simulink model "sim_att_dist_obs_tcyb"  (R2020a)
settings: Solver=ode4  StartTime=0.0  StopTime=30.0  FixedStep=0.01  RelTol=1e-3
values from neighbouring files (symbols this model uses):
  beta_Phi_1 = pp0 * cal_frac_squ( 3, p_p0_plus_1, q_p0_plus_1 )                          * cal_frac_squ( eps_s_bar / pi, p_p0_min_2, q_p0_min_2 )                          / ( 2 * ( 2 * pp0 - 1 ) * tanh( gamma0 * ( eps_s_bar / pi ) / 2 ) )                          - ( cal_frac_squ( 3, p_p0_plus_1, q_p0_plus_1 ) * gamma0 / ( 4 * ( 2 * pp0 -1 ) ) )                          * cal_frac_squ( eps_s_bar / pi, p_p0_min_ ...(+136 chars)    [init_att_dist_obs_tcyb.m]
  beta_Phi_2 = ( 1 - pp0 ) * cal_frac_squ( 3, p_p0_plus_1, q_p0_plus_1 )                          / ( 2 * ( 1 - 2 * pp0 ) * cal_frac_squ( eps_s_bar / pi, p_p0_0, q_p0_0 ) * tanh( gamma0 * ( eps_s_bar / pi ) / 2 ) )                          - ( cal_frac_squ( 3, p_p0_plus_1, q_p0_plus_1 ) * gamma0 / ( 4 * ( 1 - 2 * pp0 ) ) )                          * cal_frac_squ( eps_s_bar / pi, p_1_min_p0, q_1_min_p0 )          ...(+112 chars)    [init_att_dist_obs_tcyb.m]
  c1_diff_ui = diag([25; 30; 20])    [init_att_dist_obs_tcyb.m]
  c2_diff_ui = diag([50; 50; 10])    [init_att_dist_obs_tcyb.m]
  c3_diff_ui = diag([15; 15; 10])    [init_att_dist_obs_tcyb.m]
  c_w_1 = diag( [20; 15; 15] )    [init_att_dist_obs_tcyb.m]
  c_w_2 = diag( [20; 15; 15] )    [init_att_dist_obs_tcyb.m]
  c_w_3 = diag( [2; 2; 2] )    [init_att_dist_obs_tcyb.m]
  cS0 = diag( [4.5; 4.5; 4.5] )    [init_att_dist_obs_tcyb.m]
  dw_aa_t = 0.2 * ones(3, 5) + ( 1.0 - 0.2 ) * rand(3, 5)    [init_att_dist_obs_tcyb.m]
  dw_ff_t = [ 0.4 * ones(1, 5) + ( 1.0 - 0.4 ) * rand(1, 5);                      0.4 * ones(1, 5) + ( 1.0 - 0.4 ) * rand(1, 5);                      0.2 * ones(1, 5) + ( 0.6 - 0.2 ) * rand(1, 5) ]    [init_att_dist_obs_tcyb.m]
  dw_phi_t = ( - pi / 2 ) * ones(3, 5) + ( pi / 2 - ( - pi / 2 ) ) * rand(3, 5)    [init_att_dist_obs_tcyb.m]
  dwci_init = zeros(3,5)    [init_att_dist_obs_tcyb.m]
  eps_s_bar_div_pi = eps_s_bar / pi    (= 0.03)    [init_att_dist_obs_tcyb.m]
  gamma0 = 20    [init_att_dist_obs_tcyb.m]
  Ji = zeros(3,3,NF)    [init_att_dist_obs_tcyb.m]
  k_J_0 = diag( [1; 1; 1] )    [init_att_dist_obs_tcyb.m]
  Krw = diag([50; 50; 50])    [init_att_dist_obs_tcyb.m]
  Lamd_diff_ui = 0.8    [init_att_dist_obs_tcyb.m]
  mu_c_theta = 100    [init_att_dist_obs_tcyb.m]
  pos0 = zeros(3, 1)    [init_att_dist_obs_tcyb.m]
  pp0 = 8 / 11    (= 0.727272727273)    [init_att_dist_obs_tcyb.m]
  PZ0 = P0(3)    [init_att_dist_obs_tcyb.m]
  PZ1 = 10    [init_att_dist_obs_tcyb.m]
  Qci_init = repmat([1;0;0;0],1,NF)    [init_att_dist_obs_tcyb.m]
  R0 = 4    [init_att_dist_obs_tcyb.m]
  R1 = 8    [init_att_dist_obs_tcyb.m]
  Rci_init = zeros(3,3,NF)    [init_att_dist_obs_tcyb.m]
  Ri_init = zeros(3,3,NF)    [init_att_dist_obs_tcyb.m]
  Rx2 = 10    [init_att_dist_obs_tcyb.m]
  Ry2 = 6    [init_att_dist_obs_tcyb.m]
  Rz2 = 4    [init_att_dist_obs_tcyb.m]
  T0 = 0    [init_att_dist_obs_tcyb.m]
  T1 = tseq1    (= 10)    [init_att_dist_obs_tcyb.m]
  T2 = tseq1 + tseq12 + tseq2    (= 30)    [init_att_dist_obs_tcyb.m]
  thr_p_plus_1 = cal_frac_squ( 3, p_p0_plus_1, q_p0_plus_1 )    [init_att_dist_obs_tcyb.m]
  ui_init = zeros(3,NF)    [init_att_dist_obs_tcyb.m]
  vel0 = zeros(3, 1)    [init_att_dist_obs_tcyb.m]
  wci_init = zeros(3,5)    [init_att_dist_obs_tcyb.m]
  zeta_diff_ui = 0.05    [init_att_dist_obs_tcyb.m]
undefined symbols (not defined in the file or in its folder): cal_frac_squ, p_2_p0, p_beta_w_1, p_beta_w_2, p_p0_min_1, p_p0_plus_1, q_2_p0, q_beta_w_1, q_beta_w_2, q_p0_min_1, q_p0_plus_1, Qei_init, Qi_init, Rei_init, V_Phi_Rei_init, wei_init, wi_init
(part 2 of 4)

== matlab function sim_att_dist_obs_tcyb/Qei dynam agent 1 ==
  data: Qei_vec input; dQei_1 output; wei_vec input
function dQei_1 = fcn(Qei_vec, wei_vec)
%%%% 更新四元数误差微分方程
iiuav = 1;

wei = wei_vec(:,iiuav);
thetaei = Qei_vec(1,iiuav);
qei = Qei_vec(2:4,iiuav);

GammaQei = zeros(4,3);
GammaQei(1,:) = -(qei');
GammaQei(2:4,:) = thetaei*eye(3,3) + cal_askew_mat(qei);
dQei_1 = (1/2)*GammaQei*wei;

end

== matlab function sim_att_dist_obs_tcyb/cal d_theta_hat1 ==
  data: c1 input; d_ui_hat output; d_dui_hat output; d_d2ui_hat output; c2 input; c3 input; chi_t input; ui_sig_1 input; ui_sig_2 input; ui_sig_3 input; ui_sig_4 input; ui_sig_5 input; ui_sig_6 input; dui_hat input; d2ui_hat input
function [d_ui_hat, d_dui_hat, d_d2ui_hat] = fcn(c1, c2, c3, chi_t, ui_sig_1, ui_sig_2, ui_sig_3, ...
                                                                                        ui_sig_4, ui_sig_5, ui_sig_6, dui_hat, d2ui_hat)
d_d2ui_hat = -chi_t .* c1 * ui_sig_1(:) - (1 - chi_t) .* c1 * ui_sig_2(:);
d_dui_hat = -chi_t .* c2 * ui_sig_3(:) - (1 - chi_t) .* c2 * ui_sig_4(:) + d2ui_hat(:);
d_ui_hat = -chi_t .* c3 * ui_sig_5(:) - (1 - chi_t) .* c3 * ui_sig_6(:) + dui_hat(:);

== matlab function sim_att_dist_obs_tcyb/cal d_theta_hat2 ==
  data: c1 input; d_ui_hat output; d_dui_hat output; d_d2ui_hat output; c2 input; c3 input; chi_t input; ui_sig_1 input; ui_sig_2 input; ui_sig_3 input; ui_sig_4 input; ui_sig_5 input; ui_sig_6 input; dui_hat input; d2ui_hat input
function [d_ui_hat, d_dui_hat, d_d2ui_hat] = fcn(c1, c2, c3, chi_t, ui_sig_1, ui_sig_2, ui_sig_3, ...
                                                                                        ui_sig_4, ui_sig_5, ui_sig_6, dui_hat, d2ui_hat)
d_d2ui_hat = -chi_t .* c1 * ui_sig_1(:) - (1 - chi_t) .* c1 * ui_sig_2(:);
d_dui_hat = -chi_t .* c2 * ui_sig_3(:) - (1 - chi_t) .* c2 * ui_sig_4(:) + d2ui_hat(:);
d_ui_hat = -chi_t .* c3 * ui_sig_5(:) - (1 - chi_t) .* c3 * ui_sig_6(:) + dui_hat(:);

== matlab function sim_att_dist_obs_tcyb/cal d_theta_hat3 ==
  data: c1 input; d_ui_hat output; d_dui_hat output; d_d2ui_hat output; c2 input; c3 input; chi_t input; ui_sig_1 input; ui_sig_2 input; ui_sig_3 input; ui_sig_4 input; ui_sig_5 input; ui_sig_6 input; dui_hat input; d2ui_hat input
function [d_ui_hat, d_dui_hat, d_d2ui_hat] = fcn(c1, c2, c3, chi_t, ui_sig_1, ui_sig_2, ui_sig_3, ...
                                                                                        ui_sig_4, ui_sig_5, ui_sig_6, dui_hat, d2ui_hat)
d_d2ui_hat = -chi_t .* c1 * ui_sig_1(:) - (1 - chi_t) .* c1 * ui_sig_2(:);
d_dui_hat = -chi_t .* c2 * ui_sig_3(:) - (1 - chi_t) .* c2 * ui_sig_4(:) + d2ui_hat(:);
d_ui_hat = -chi_t .* c3 * ui_sig_5(:) - (1 - chi_t) .* c3 * ui_sig_6(:) + dui_hat(:);

== matlab function sim_att_dist_obs_tcyb/cal d_theta_hat4 ==
  data: c1 input; d_ui_hat output; d_dui_hat output; d_d2ui_hat output; c2 input; c3 input; chi_t input; ui_sig_1 input; ui_sig_2 input; ui_sig_3 input; ui_sig_4 input; ui_sig_5 input; ui_sig_6 input; dui_hat input; d2ui_hat input
function [d_ui_hat, d_dui_hat, d_d2ui_hat] = fcn(c1, c2, c3, chi_t, ui_sig_1, ui_sig_2, ui_sig_3, ...
                                                                                        ui_sig_4, ui_sig_5, ui_sig_6, dui_hat, d2ui_hat)
d_d2ui_hat = -chi_t .* c1 * ui_sig_1(:) - (1 - chi_t) .* c1 * ui_sig_2(:);
d_dui_hat = -chi_t .* c2 * ui_sig_3(:) - (1 - chi_t) .* c2 * ui_sig_4(:) + d2ui_hat(:);
d_ui_hat = -chi_t .* c3 * ui_sig_5(:) - (1 - chi_t) .* c3 * ui_sig_6(:) + dui_hat(:);

== matlab function sim_att_dist_obs_tcyb/process velocity ==
  data: T0 input; T1 input; T2 input; PZ0 input; PZ1 input; R0 input; R1 input; Rx2 input; Ry2 input; Rz2 input; t input; V_init_out output
function V_init_out = fcn(T0, T1, T2, PZ0, PZ1, R0, R1, Rx2, Ry2, Rz2, t)
V_init_out = zeros(3, 1);
if t < T1 + 1e-05
    V_init_out(1, 1) = ( cos( ( 2 * pi * ( t - T0 ) ) / ( T0 - T1 ) ) * ( R0 - R1 ) ) / ( T0 - T1 ) ...
                                    - ( 2 * pi * sin( ( 2 * pi * ( t - T0 ) ) / ( T0 - T1 ) ) * ( R0 + ( ( R0 - R1 ) * ( t - T0 ) ) / ( T0 - T1 ) ) ) / ( T0 - T1 );
    V_init_out(2, 1) = ( sin( ( 2 * pi * ( t - T0 ) ) / ( T0 - T1 ) ) * ( R0 - R1 ) ) / ( T0 - T1 ) ...
                                    + ( 2 * pi * cos( ( 2 * pi * ( t - T0 ) ) / ( T0 - T1 ) ) * ( R0 + ( ( R0 - R1 ) * ( t - T0 ) ) / ( T0 - T1 ) ) ) / ( T0 - T1 );
    V_init_out(3, 1) = ( PZ0 - PZ1 ) / ( T0 - T1 );
else
    V_init_out(1, 1) = ( 2 * Rx2 * pi * sin( ( 2 * pi * ( t - T1 ) ) / ( T1 - T2 ) ) ) / ( T1 - T2 );
    V_init_out(2, 1) = ( 4 * Ry2 * pi * cos( ( 4 * pi * ( t - T1 ) ) / ( T1 - T2 ) ) ) / ( T1 - T2 );
    V_init_out(3, 1) = - ( 4 * Rz2 * pi * cos( ( 4 * pi * ( t - T1 ) ) / ( T1 - T2 ) ) ) / ( T1 - T2 );
end

== matlab function sim_att_dist_obs_tcyb/cal divide pi ==
  data: x input; y output
function y = fcn(x)
y = x ./ pi;

== matlab function sim_att_dist_obs_tcyb/cal sig ==
  data: x input; z output; y input
function z = fcn(x, y)
z = x(:) .* sign(y(:));

== matlab function sim_att_dist_obs_tcyb/cal sig1 ==
  data: x input; z output; y input
function z = fcn(x, y)
z = x(:) .* sign(y(:));

== matlab function sim_att_dist_obs_tcyb/cal sig10 ==
  data: x input; z output; y input
function z = fcn(x, y)
z = x(:) .* sign(y(:));

== matlab function sim_att_dist_obs_tcyb/cal sig11 ==
  data: x input; z output; y input
function z = fcn(x, y)
z = x(:) .* sign(y(:));

== matlab function sim_att_dist_obs_tcyb/cal sig12 ==
  data: x input; z output; y input
function z = fcn(x, y)
z = x(:) .* sign(y(:));

== matlab function sim_att_dist_obs_tcyb/cal sig13 ==
  data: x input; z output; y input
function z = fcn(x, y)
z = x(:) .* sign(y(:));

== matlab function sim_att_dist_obs_tcyb/cal sig14 ==
  data: x input; z output; y input
function z = fcn(x, y)
z = x(:) .* sign(y(:));

== matlab function sim_att_dist_obs_tcyb/cal sig15 ==
  data: x input; z output; y input
function z = fcn(x, y)
z = x(:) .* sign(y(:));

== matlab function sim_att_dist_obs_tcyb/cal sig16 ==
  data: x input; z output; y input
function z = fcn(x, y)
z = x(:) .* sign(y(:));

== matlab function sim_att_dist_obs_tcyb/cal sig17 ==
  data: x input; z output; y input
function z = fcn(x, y)
z = x(:) .* sign(y(:));

== matlab function sim_att_dist_obs_tcyb/cal sig18 ==
  data: x input; z output; y input
function z = fcn(x, y)
z = x(:) .* sign(y(:));

== matlab function sim_att_dist_obs_tcyb/cal sig19 ==
  data: x input; z output; y input
function z = fcn(x, y)
z = x(:) .* sign(y(:));

== matlab function sim_att_dist_obs_tcyb/cal sig2 ==
  data: x input; z output; y input
function z = fcn(x, y)
z = x(:) .* sign(y(:));

== matlab function sim_att_dist_obs_tcyb/cal sig20 ==
  data: x input; z output; y input
function z = fcn(x, y)
z = x(:) .* sign(y(:));

== matlab function sim_att_dist_obs_tcyb/cal sig21 ==
  data: x input; z output; y input
function z = fcn(x, y)
z = x(:) .* sign(y(:));

== matlab function sim_att_dist_obs_tcyb/cal sig22 ==
  data: x input; z output; y input
function z = fcn(x, y)
z = x(:) .* sign(y(:));

== matlab function sim_att_dist_obs_tcyb/cal sig23 ==
  data: x input; z output; y input
function z = fcn(x, y)
z = x(:) .* sign(y(:));

== matlab function sim_att_dist_obs_tcyb/cal sig24 ==
  data: x input; z output; y input
function z = fcn(x, y)
z = x(:) .* sign(y(:));

== matlab function sim_att_dist_obs_tcyb/cal sig25 ==
  data: x input; z output; y input
function z = fcn(x, y)
z = x(:) .* sign(y(:));

== matlab function sim_att_dist_obs_tcyb/cal sig26 ==
  data: x input; z output; y input
function z = fcn(x, y)
z = x(:) .* sign(y(:));

== matlab function sim_att_dist_obs_tcyb/Qei dynam agent 2 ==
  data: Qei_vec input; dQei_2 output; wei_vec input
function dQei_2 = fcn(Qei_vec, wei_vec)
%%%% 更新四元数误差微分方程
iiuav = 2;

wei = wei_vec(:,iiuav);
thetaei = Qei_vec(1,iiuav);
qei = Qei_vec(2:4,iiuav);

GammaQei = zeros(4,3);
GammaQei(1,:) = -(qei');
GammaQei(2:4,:) = thetaei*eye(3,3) + cal_askew_mat(qei);
dQei_2 = (1/2)*GammaQei*wei;

end

== matlab function sim_att_dist_obs_tcyb/cal sig27 ==
  data: x input; z output; y input
function z = fcn(x, y)
z = x(:) .* sign(y(:));

== matlab function sim_att_dist_obs_tcyb/cal sig28 ==
  data: x input; z output; y input
function z = fcn(x, y)
z = x(:) .* sign(y(:));

== matlab function sim_att_dist_obs_tcyb/cal sig29 ==
  data: x input; z output; y input
function z = fcn(x, y)
z = x(:) .* sign(y(:));

== matlab function sim_att_dist_obs_tcyb/cal sig3 ==
  data: x input; z output; y input
function z = fcn(x, y)
z = x(:) .* sign(y(:));

== matlab function sim_att_dist_obs_tcyb/cal sig4 ==
  data: x input; z output; y input
function z = fcn(x, y)
z = x(:) .* sign(y(:));

== matlab function sim_att_dist_obs_tcyb/cal sig5 ==
  data: x input; z output; y input
function z = fcn(x, y)
z = x(:) .* sign(y(:));

== matlab function sim_att_dist_obs_tcyb/cal sig6 ==
  data: x input; z output; y input
function z = fcn(x, y)
z = x(:) .* sign(y(:));

== matlab function sim_att_dist_obs_tcyb/cal sig7 ==
  data: x input; z output; y input
function z = fcn(x, y)
z = x(:) .* sign(y(:));

== matlab function sim_att_dist_obs_tcyb/cal sig8 ==
  data: x input; z output; y input
function z = fcn(x, y)
z = x(:) .* sign(y(:));

== matlab function sim_att_dist_obs_tcyb/cal sig9 ==
  data: x input; z output; y input
function z = fcn(x, y)
z = x(:) .* sign(y(:));

== matlab function sim_att_dist_obs_tcyb/combine dw_hat1 ==
  data: eps_w_hat_1 input; eps_w_hat_2 input; eps_w_hat_3 input; eps_w_hat_4 input; eps_w_hat_5 input; eps_w_hat_vec output
function eps_w_hat_vec  = fcn(eps_w_hat_1, eps_w_hat_2, eps_w_hat_3, eps_w_hat_4, eps_w_hat_5)
%%%% 合并扰动观测值dw_hat
eps_w_hat_vec = [eps_w_hat_1(:), eps_w_hat_2(:), eps_w_hat_3(:), eps_w_hat_4(:), eps_w_hat_5(:)];

== matlab function sim_att_dist_obs_tcyb/cal taui agent 1 ==
  data: c_w_1 input; c_w_2 input; c_w_3 input; k_J_0 input; tau_1 output; Ji input; Si_vec input; dw_hat_vec input; Fi_S_vec input; theta_Si_beta_w_1_vec input; theta_Si_beta_w_2_vec input
function tau_1 = fcn(c_w_1, c_w_2, c_w_3, k_J_0, Ji, Si_vec, dw_hat_vec, ...
                                        Fi_S_vec, theta_Si_beta_w_1_vec, theta_Si_beta_w_2_vec)
%%%% 计算用于姿态控制的驱动力矩控制输入
iiuav = 1;
tau_1 = -c_w_1 * theta_Si_beta_w_1_vec(:,iiuav) - c_w_2 * theta_Si_beta_w_2_vec(:,iiuav) - c_w_3 * Si_vec(:,iiuav) ...
                - dw_hat_vec(:,iiuav) - k_J_0 * inv( Ji(:,:,iiuav) ) * Fi_S_vec(:,iiuav);
end

== matlab function sim_att_dist_obs_tcyb/cal taui agent 2 ==
  data: c_w_1 input; c_w_2 input; c_w_3 input; k_J_0 input; tau_2 output; Ji input; Si_vec input; dw_hat_vec input; Fi_S_vec input; theta_Si_beta_w_1_vec input; theta_Si_beta_w_2_vec input
function tau_2 = fcn(c_w_1, c_w_2, c_w_3, k_J_0, Ji, Si_vec, dw_hat_vec, ...
                                        Fi_S_vec, theta_Si_beta_w_1_vec, theta_Si_beta_w_2_vec)
%%%% 计算用于姿态控制的驱动力矩控制输入
iiuav = 2;
tau_2 = -c_w_1 * theta_Si_beta_w_1_vec(:,iiuav) - c_w_2 * theta_Si_beta_w_2_vec(:,iiuav) - c_w_3 * Si_vec(:,iiuav) ...
                - dw_hat_vec(:,iiuav) - k_J_0 * inv( Ji(:,:,iiuav) ) * Fi_S_vec(:,iiuav);
end

== matlab function sim_att_dist_obs_tcyb/cal taui agent 3 ==
  data: c_w_1 input; c_w_2 input; c_w_3 input; k_J_0 input; tau_3 output; Ji input; Si_vec input; dw_hat_vec input; Fi_S_vec input; theta_Si_beta_w_1_vec input; theta_Si_beta_w_2_vec input
function tau_3 = fcn(c_w_1, c_w_2, c_w_3, k_J_0, Ji, Si_vec, dw_hat_vec, ...
                                        Fi_S_vec, theta_Si_beta_w_1_vec, theta_Si_beta_w_2_vec)
%%%% 计算用于姿态控制的驱动力矩控制输入
iiuav = 3;
tau_3 = -c_w_1 * theta_Si_beta_w_1_vec(:,iiuav) - c_w_2 * theta_Si_beta_w_2_vec(:,iiuav) - c_w_3 * Si_vec(:,iiuav) ...
                - dw_hat_vec(:,iiuav) - k_J_0 * inv( Ji(:,:,iiuav) ) * Fi_S_vec(:,iiuav);
end

== matlab function sim_att_dist_obs_tcyb/cal taui agent 4 ==
  data: c_w_1 input; c_w_2 input; c_w_3 input; k_J_0 input; tau_4 output; Ji input; Si_vec input; dw_hat_vec input; Fi_S_vec input; theta_Si_beta_w_1_vec input; theta_Si_beta_w_2_vec input
function tau_4 = fcn(c_w_1, c_w_2, c_w_3, k_J_0, Ji, Si_vec, dw_hat_vec, ...
                                        Fi_S_vec, theta_Si_beta_w_1_vec, theta_Si_beta_w_2_vec)
%%%% 计算用于姿态控制的驱动力矩控制输入
iiuav = 4;
tau_4 = -c_w_1 * theta_Si_beta_w_1_vec(:,iiuav) - c_w_2 * theta_Si_beta_w_2_vec(:,iiuav) - c_w_3 * Si_vec(:,iiuav) ...
                - dw_hat_vec(:,iiuav) - k_J_0 * inv( Ji(:,:,iiuav) ) * Fi_S_vec(:,iiuav);
end

== matlab function sim_att_dist_obs_tcyb/cal taui agent 5 ==
  data: c_w_1 input; c_w_2 input; c_w_3 input; k_J_0 input; tau_5 output; Ji input; Si_vec input; dw_hat_vec input; Fi_S_vec input; theta_Si_beta_w_1_vec input; theta_Si_beta_w_2_vec input
function tau_5 = fcn(c_w_1, c_w_2, c_w_3, k_J_0, Ji, Si_vec, dw_hat_vec, ...
                                        Fi_S_vec, theta_Si_beta_w_1_vec, theta_Si_beta_w_2_vec)
%%%% 计算用于姿态控制的驱动力矩控制输入
iiuav = 5;
tau_5 = -c_w_1 * theta_Si_beta_w_1_vec(:,iiuav) - c_w_2 * theta_Si_beta_w_2_vec(:,iiuav) - c_w_3 * Si_vec(:,iiuav) ...
                - dw_hat_vec(:,iiuav) - k_J_0 * inv( Ji(:,:,iiuav) ) * Fi_S_vec(:,iiuav);
end

== matlab function sim_att_dist_obs_tcyb/cal theta_Si_beta_w agent 1 ==
  data: mu_c_theta input; Si_squ_beta_w_1_vec input; theta_Si_beta_w_1_node_1 output; Si_squ_beta_w_2_vec input; Si_vec input; theta_Si_beta_w_2_node_1 output
function [theta_Si_beta_w_1_node_1, theta_Si_beta_w_2_node_1] = fcn(mu_c_theta, Si_squ_beta_w_1_vec, Si_squ_beta_w_2_vec, Si_vec)
%%%% 计算平滑递增函数
iiuav = 1;
theta_Si_beta_w_1_node_1 = Si_squ_beta_w_1_vec(:, iiuav) .* ( -1 + 2 ./ ( 1 + exp( -mu_c_theta .* Si_vec(:,iiuav) ) ) );
theta_Si_beta_w_2_node_1 = Si_squ_beta_w_2_vec(:, iiuav) .* ( -1 + 2 ./ ( 1 + exp( -mu_c_theta .* Si_vec(:,iiuav) ) ) );

== matlab function sim_att_dist_obs_tcyb/cal theta_Si_beta_w agent 2 ==
  data: mu_c_theta input; Si_squ_beta_w_1_vec input; theta_Si_beta_w_1_node_2 output; Si_squ_beta_w_2_vec input; Si_vec input; theta_Si_beta_w_2_node_2 output
function [theta_Si_beta_w_1_node_2, theta_Si_beta_w_2_node_2] = fcn(mu_c_theta, Si_squ_beta_w_1_vec, Si_squ_beta_w_2_vec, Si_vec)
%%%% 计算平滑递增函数
iiuav = 2;
theta_Si_beta_w_1_node_2 = Si_squ_beta_w_1_vec(:, iiuav) .* ( -1 + 2 ./ ( 1 + exp( -mu_c_theta .* Si_vec(:,iiuav) ) ) );
theta_Si_beta_w_2_node_2 = Si_squ_beta_w_2_vec(:, iiuav) .* ( -1 + 2 ./ ( 1 + exp( -mu_c_theta .* Si_vec(:,iiuav) ) ) );

== matlab function sim_att_dist_obs_tcyb/cal theta_Si_beta_w agent 3 ==
  data: mu_c_theta input; Si_squ_beta_w_1_vec input; theta_Si_beta_w_1_node_3 output; Si_squ_beta_w_2_vec input; Si_vec input; theta_Si_beta_w_2_node_3 output
function [theta_Si_beta_w_1_node_3, theta_Si_beta_w_2_node_3] = fcn(mu_c_theta, Si_squ_beta_w_1_vec, Si_squ_beta_w_2_vec, Si_vec)
%%%% 计算平滑递增函数
iiuav = 3;
theta_Si_beta_w_1_node_3 = Si_squ_beta_w_1_vec(:, iiuav) .* ( -1 + 2 ./ ( 1 + exp( -mu_c_theta .* Si_vec(:,iiuav) ) ) );
theta_Si_beta_w_2_node_3 = Si_squ_beta_w_2_vec(:, iiuav) .* ( -1 + 2 ./ ( 1 + exp( -mu_c_theta .* Si_vec(:,iiuav) ) ) );

== matlab function sim_att_dist_obs_tcyb/cal eps_w_hat agent 1 ==
  data: Ji input; Krw input; eps_w_hat_vec input; wi_vec input; d_eps_w_hat_1 output; taui_vec input
function d_eps_w_hat_1 = fcn(Ji, Krw, eps_w_hat_vec, wi_vec, taui_vec)
%%%% 计算扰动观测中间变量
iiuav = 1;
d_eps_w_hat_1 = -Krw * inv(Ji(:,:,iiuav)) * ( eps_w_hat_vec(:,iiuav) + taui_vec(:,iiuav) ...
                                                                        - cal_askew_mat(wi_vec(:,iiuav)) * Ji(:,:,iiuav) * wi_vec(:,iiuav) ) ...
                                                                        - Krw * Krw * inv(Ji(:,:,iiuav)) * wi_vec(:,iiuav);

== matlab function sim_att_dist_obs_tcyb/cal theta_Si_beta_w agent 4 ==
  data: mu_c_theta input; Si_squ_beta_w_1_vec input; theta_Si_beta_w_1_node_4 output; Si_squ_beta_w_2_vec input; Si_vec input; theta_Si_beta_w_2_node_4 output
function [theta_Si_beta_w_1_node_4, theta_Si_beta_w_2_node_4] = fcn(mu_c_theta, Si_squ_beta_w_1_vec, Si_squ_beta_w_2_vec, Si_vec)
%%%% 计算平滑递增函数
iiuav = 4;
theta_Si_beta_w_1_node_4 = Si_squ_beta_w_1_vec(:, iiuav) .* ( -1 + 2 ./ ( 1 + exp( -mu_c_theta .* Si_vec(:,iiuav) ) ) );
theta_Si_beta_w_2_node_4 = Si_squ_beta_w_2_vec(:, iiuav) .* ( -1 + 2 ./ ( 1 + exp( -mu_c_theta .* Si_vec(:,iiuav) ) ) );

== matlab function sim_att_dist_obs_tcyb/cal theta_Si_beta_w agent 5 ==
  data: mu_c_theta input; Si_squ_beta_w_1_vec input; theta_Si_beta_w_1_node_5 output; Si_squ_beta_w_2_vec input; Si_vec input; theta_Si_beta_w_2_node_5 output
function [theta_Si_beta_w_1_node_5, theta_Si_beta_w_2_node_5] = fcn(mu_c_theta, Si_squ_beta_w_1_vec, Si_squ_beta_w_2_vec, Si_vec)
%%%% 计算平滑递增函数
iiuav = 5;
theta_Si_beta_w_1_node_5 = Si_squ_beta_w_1_vec(:, iiuav) .* ( -1 + 2 ./ ( 1 + exp( -mu_c_theta .* Si_vec(:,iiuav) ) ) );
theta_Si_beta_w_2_node_5 = Si_squ_beta_w_2_vec(:, iiuav) .* ( -1 + 2 ./ ( 1 + exp( -mu_c_theta .* Si_vec(:,iiuav) ) ) );

== matlab function sim_att_dist_obs_tcyb/cal wci dwci agent 1 ==
  data: ui_vec input; wci output; duihat_vec input; d2uihat_vec input; Rci_mat input; dwci output
function [wci, dwci] = fcn(ui_vec, duihat_vec, d2uihat_vec, Rci_mat)
%%%% 计算姿态角速率指令及其导数

iiuav = 1;
ui = ui_vec(:,iiuav);
duihat = duihat_vec(:,iiuav);
d2uihat = d2uihat_vec(:,iiuav);
Rci = Rci_mat(:,:,iiuav);

ee1 = [1;0;0];
ee2 = [0;1;0];
ee3 = [0;0;1];
RciE3 = ui / norm(ui,2);
PiMat = eye(3,3) - ee3*(ee3');
dRciE3 = (1 / norm(ui,2))*Rci*PiMat*(Rci')*duihat;
Themat = [-RciE3(2)/(1+RciE3(3)),         -RciE3(1)/(1+RciE3(3)),       (RciE3(1)*RciE3(2))/((1+RciE3(3))^2); ...
                   2*RciE3(1)/(1+RciE3(3)),                0,                               1 - (RciE3(1)^2)/((1+RciE3(3))^2); ...
                               0                                       -1                                                        0                                   ];
wcxe3 = (1 / norm(ui,2))*PiMat*(Rci')*duihat;
wcxe2 = (1 / norm(ui,2))*(Rci')*Themat*Rci*PiMat*(Rci')*duihat;
wci = [-wcxe3(2); wcxe3(1); -wcxe2(1)];

TempMat1 = [0,                           -1/(1+RciE3(3)),                   (RciE3(2))/((1+RciE3(3))^2); ...
                       2/(1+RciE3(3)),                0,                               (-2*RciE3(1))/((1+RciE3(3))^2); ...
                       0,                                     0,                                                   0                             ];
TempMat2 = [-1/(1+RciE3(3)),              0,                               (RciE3(1))/((1+RciE3(3))^2); ...
                       0,                                     0,                                                   0                      ; ...
                       0,                                     0,                                                   0                             ];
TempMat3 = [(RciE3(2))/((1+RciE3(3))^2),                 (RciE3(1))/((1+RciE3(3))^2),       (-2*RciE3(1)*RciE3(2))/((1+RciE3(3))^3); ...
                       (-2*RciE3(1))/((1+RciE3(3))^2),                             0,                               (2*(RciE3(1)^2))/((1+RciE3(3))^3); ...
                        0,                                                                          0,                                                   0                             ];
dTheMat = TempMat1*dRciE3*(ee1') + TempMat2*dRciE3*(ee2') + TempMat3*dRciE3*(ee3');
wcix = cal_askew_mat(wci);
dRciT = -wcix*(Rci');
dwcxe3 = (1 / norm(ui,2))*PiMat*(dRciT*duihat+(Rci')*(d2uihat-(((ui')*duihat)/(norm(ui,2)^2))*duihat));
dwcxe2 = (1 / norm(ui,2))*((dRciT*Themat+(Rci')*dTheMat) ...
                *(Rci*PiMat*(Rci'))*duihat + (Rci')*Themat*(Rci*PiMat*(Rci'))*(d2uihat-(((ui')*duihat)/(norm(ui,2)^2))*duihat));
dwci = [-dwcxe3(2);  dwcxe3(1);  -dwcxe2(1)];

== matlab function sim_att_dist_obs_tcyb/cal wci dwci agent 2 ==
  data: ui_vec input; wci output; duihat_vec input; d2uihat_vec input; Rci_mat input; dwci output
function [wci, dwci] = fcn(ui_vec, duihat_vec, d2uihat_vec, Rci_mat)
%%%% 计算姿态角速率指令及其导数

iiuav = 2;
ui = ui_vec(:,iiuav);
duihat = duihat_vec(:,iiuav);
d2uihat = d2uihat_vec(:,iiuav);
Rci = Rci_mat(:,:,iiuav);

ee1 = [1;0;0];
ee2 = [0;1;0];
ee3 = [0;0;1];
RciE3 = ui / norm(ui,2);
PiMat = eye(3,3) - ee3*(ee3');
dRciE3 = (1 / norm(ui,2))*Rci*PiMat*(Rci')*duihat;
Themat = [-RciE3(2)/(1+RciE3(3)),         -RciE3(1)/(1+RciE3(3)),       (RciE3(1)*RciE3(2))/((1+RciE3(3))^2); ...
                   2*RciE3(1)/(1+RciE3(3)),                0,                               1 - (RciE3(1)^2)/((1+RciE3(3))^2); ...
                               0                                       -1                                                        0                                   ];
wcxe3 = (1 / norm(ui,2))*PiMat*(Rci')*duihat;
wcxe2 = (1 / norm(ui,2))*(Rci')*Themat*Rci*PiMat*(Rci')*duihat;
wci = [-wcxe3(2); wcxe3(1); -wcxe2(1)];

TempMat1 = [0,                           -1/(1+RciE3(3)),                   (RciE3(2))/((1+RciE3(3))^2); ...
                       2/(1+RciE3(3)),                0,                               (-2*RciE3(1))/((1+RciE3(3))^2); ...
                       0,                                     0,                                                   0                             ];
TempMat2 = [-1/(1+RciE3(3)),              0,                               (RciE3(1))/((1+RciE3(3))^2); ...
                       0,                                     0,                                                   0                      ; ...
                       0,                                     0,                                                   0                             ];
TempMat3 = [(RciE3(2))/((1+RciE3(3))^2),                 (RciE3(1))/((1+RciE3(3))^2),       (-2*RciE3(1)*RciE3(2))/((1+RciE3(3))^3); ...
                       (-2*RciE3(1))/((1+RciE3(3))^2),                             0,                               (2*(RciE3(1)^2))/((1+RciE3(3))^3); ...
                        0,                                                                          0,                                                   0                             ];
dTheMat = TempMat1*dRciE3*(ee1') + TempMat2*dRciE3*(ee2') + TempMat3*dRciE3*(ee3');
wcix = cal_askew_mat(wci);
dRciT = -wcix*(Rci');
dwcxe3 = (1 / norm(ui,2))*PiMat*(dRciT*duihat+(Rci')*(d2uihat-(((ui')*duihat)/(norm(ui,2)^2))*duihat));
dwcxe2 = (1 / norm(ui,2))*((dRciT*Themat+(Rci')*dTheMat) ...
                *(Rci*PiMat*(Rci'))*duihat + (Rci')*Themat*(Rci*PiMat*(Rci'))*(d2uihat-(((ui')*duihat)/(norm(ui,2)^2))*duihat));
dwci = [-dwcxe3(2);  dwcxe3(1);  -dwcxe2(1)];

== matlab function sim_att_dist_obs_tcyb/cal wci dwci agent 3 ==
  data: ui_vec input; wci output; duihat_vec input; d2uihat_vec input; Rci_mat input; dwci output
function [wci, dwci] = fcn(ui_vec, duihat_vec, d2uihat_vec, Rci_mat)
%%%% 计算姿态角速率指令及其导数

iiuav = 3;
ui = ui_vec(:,iiuav);
duihat = duihat_vec(:,iiuav);
d2uihat = d2uihat_vec(:,iiuav);
Rci = Rci_mat(:,:,iiuav);

ee1 = [1;0;0];
ee2 = [0;1;0];
ee3 = [0;0;1];
RciE3 = ui / norm(ui,2);
PiMat = eye(3,3) - ee3*(ee3');
dRciE3 = (1 / norm(ui,2))*Rci*PiMat*(Rci')*duihat;
Themat = [-RciE3(2)/(1+RciE3(3)),         -RciE3(1)/(1+RciE3(3)),       (RciE3(1)*RciE3(2))/((1+RciE3(3))^2); ...
                   2*RciE3(1)/(1+RciE3(3)),                0,                               1 - (RciE3(1)^2)/((1+RciE3(3))^2); ...
                               0                                       -1                                                        0                                   ];
wcxe3 = (1 / norm(ui,2))*PiMat*(Rci')*duihat;
wcxe2 = (1 / norm(ui,2))*(Rci')*Themat*Rci*PiMat*(Rci')*duihat;
wci = [-wcxe3(2); wcxe3(1); -wcxe2(1)];

TempMat1 = [0,                           -1/(1+RciE3(3)),                   (RciE3(2))/((1+RciE3(3))^2); ...
                       2/(1+RciE3(3)),                0,                               (-2*RciE3(1))/((1+RciE3(3))^2); ...
                       0,                                     0,                                                   0                             ];
TempMat2 = [-1/(1+RciE3(3)),              0,                               (RciE3(1))/((1+RciE3(3))^2); ...
                       0,                                     0,                                                   0                      ; ...
                       0,                                     0,                                                   0                             ];
TempMat3 = [(RciE3(2))/((1+RciE3(3))^2),                 (RciE3(1))/((1+RciE3(3))^2),       (-2*RciE3(1)*RciE3(2))/((1+RciE3(3))^3); ...
                       (-2*RciE3(1))/((1+RciE3(3))^2),                             0,                               (2*(RciE3(1)^2))/((1+RciE3(3))^3); ...
                        0,                                                                          0,                                                   0                             ];
dTheMat = TempMat1*dRciE3*(ee1') + TempMat2*dRciE3*(ee2') + TempMat3*dRciE3*(ee3');
wcix = cal_askew_mat(wci);
dRciT = -wcix*(Rci');
dwcxe3 = (1 / norm(ui,2))*PiMat*(dRciT*duihat+(Rci')*(d2uihat-(((ui')*duihat)/(norm(ui,2)^2))*duihat));
dwcxe2 = (1 / norm(ui,2))*((dRciT*Themat+(Rci')*dTheMat) ...
                *(Rci*PiMat*(Rci'))*duihat + (Rci')*Themat*(Rci*PiMat*(Rci'))*(d2uihat-(((ui')*duihat)/(norm(ui,2)^2))*duihat));
dwci = [-dwcxe3(2);  dwcxe3(1);  -dwcxe2(1)];

== matlab function sim_att_dist_obs_tcyb/cal wci dwci agent 4 ==
  data: ui_vec input; wci output; duihat_vec input; d2uihat_vec input; Rci_mat input; dwci output
function [wci, dwci] = fcn(ui_vec, duihat_vec, d2uihat_vec, Rci_mat)
%%%% 计算姿态角速率指令及其导数

iiuav = 4;
ui = ui_vec(:,iiuav);
duihat = duihat_vec(:,iiuav);
d2uihat = d2uihat_vec(:,iiuav);
Rci = Rci_mat(:,:,iiuav);

ee1 = [1;0;0];
ee2 = [0;1;0];
ee3 = [0;0;1];
RciE3 = ui / norm(ui,2);
PiMat = eye(3,3) - ee3*(ee3');
dRciE3 = (1 / norm(ui,2))*Rci*PiMat*(Rci')*duihat;
Themat = [-RciE3(2)/(1+RciE3(3)),         -RciE3(1)/(1+RciE3(3)),       (RciE3(1)*RciE3(2))/((1+RciE3(3))^2); ...
                   2*RciE3(1)/(1+RciE3(3)),                0,                               1 - (RciE3(1)^2)/((1+RciE3(3))^2); ...
                               0                                       -1                                                        0                                   ];
wcxe3 = (1 / norm(ui,2))*PiMat*(Rci')*duihat;
wcxe2 = (1 / norm(ui,2))*(Rci')*Themat*Rci*PiMat*(Rci')*duihat;
wci = [-wcxe3(2); wcxe3(1); -wcxe2(1)];

TempMat1 = [0,                           -1/(1+RciE3(3)),                   (RciE3(2))/((1+RciE3(3))^2); ...
                       2/(1+RciE3(3)),                0,                               (-2*RciE3(1))/((1+RciE3(3))^2); ...
                       0,                                     0,                                                   0                             ];
TempMat2 = [-1/(1+RciE3(3)),              0,                               (RciE3(1))/((1+RciE3(3))^2); ...
                       0,                                     0,                                                   0                      ; ...
                       0,                                     0,                                                   0                             ];
TempMat3 = [(RciE3(2))/((1+RciE3(3))^2),                 (RciE3(1))/((1+RciE3(3))^2),       (-2*RciE3(1)*RciE3(2))/((1+RciE3(3))^3); ...
                       (-2*RciE3(1))/((1+RciE3(3))^2),                             0,                               (2*(RciE3(1)^2))/((1+RciE3(3))^3); ...
                        0,                                                                          0,                                                   0                             ];
dTheMat = TempMat1*dRciE3*(ee1') + TempMat2*dRciE3*(ee2') + TempMat3*dRciE3*(ee3');
wcix = cal_askew_mat(wci);
dRciT = -wcix*(Rci');
dwcxe3 = (1 / norm(ui,2))*PiMat*(dRciT*duihat+(Rci')*(d2uihat-(((ui')*duihat)/(norm(ui,2)^2))*duihat));
dwcxe2 = (1 / norm(ui,2))*((dRciT*Themat+(Rci')*dTheMat) ...
                *(Rci*PiMat*(Rci'))*duihat + (Rci')*Themat*(Rci*PiMat*(Rci'))*(d2uihat-(((ui')*duihat)/(norm(ui,2)^2))*duihat));
dwci = [-dwcxe3(2);  dwcxe3(1);  -dwcxe2(1)];

== matlab function sim_att_dist_obs_tcyb/cal wci dwci agent 5 ==
  data: ui_vec input; wci output; duihat_vec input; d2uihat_vec input; Rci_mat input; dwci output
function [wci, dwci] = fcn(ui_vec, duihat_vec, d2uihat_vec, Rci_mat)
%%%% 计算姿态角速率指令及其导数

iiuav = 5;
ui = ui_vec(:,iiuav);
duihat = duihat_vec(:,iiuav);
d2uihat = d2uihat_vec(:,iiuav);
Rci = Rci_mat(:,:,iiuav);

ee1 = [1;0;0];
ee2 = [0;1;0];
ee3 = [0;0;1];
RciE3 = ui / norm(ui,2);
PiMat = eye(3,3) - ee3*(ee3');
dRciE3 = (1 / norm(ui,2))*Rci*PiMat*(Rci')*duihat;
Themat = [-RciE3(2)/(1+RciE3(3)),         -RciE3(1)/(1+RciE3(3)),       (RciE3(1)*RciE3(2))/((1+RciE3(3))^2); ...
                   2*RciE3(1)/(1+RciE3(3)),                0,                               1 - (RciE3(1)^2)/((1+RciE3(3))^2); ...
                               0                                       -1                                                        0                                   ];
wcxe3 = (1 / norm(ui,2))*PiMat*(Rci')*duihat;
wcxe2 = (1 / norm(ui,2))*(Rci')*Themat*Rci*PiMat*(Rci')*duihat;
wci = [-wcxe3(2); wcxe3(1); -wcxe2(1)];

TempMat1 = [0,                           -1/(1+RciE3(3)),                   (RciE3(2))/((1+RciE3(3))^2); ...
                       2/(1+RciE3(3)),                0,                               (-2*RciE3(1))/((1+RciE3(3))^2); ...
                       0,                                     0,                                                   0                             ];
TempMat2 = [-1/(1+RciE3(3)),              0,                               (RciE3(1))/((1+RciE3(3))^2); ...
                       0,                                     0,                                                   0                      ; ...
                       0,                                     0,                                                   0                             ];
TempMat3 = [(RciE3(2))/((1+RciE3(3))^2),                 (RciE3(1))/((1+RciE3(3))^2),       (-2*RciE3(1)*RciE3(2))/((1+RciE3(3))^3); ...
                       (-2*RciE3(1))/((1+RciE3(3))^2),                             0,                               (2*(RciE3(1)^2))/((1+RciE3(3))^3); ...
                        0,                                                                          0,                                                   0                             ];
dTheMat = TempMat1*dRciE3*(ee1') + TempMat2*dRciE3*(ee2') + TempMat3*dRciE3*(ee3');
wcix = cal_askew_mat(wci);
dRciT = -wcix*(Rci');
dwcxe3 = (1 / norm(ui,2))*PiMat*(dRciT*duihat+(Rci')*(d2uihat-(((ui')*duihat)/(norm(ui,2)^2))*duihat));
dwcxe2 = (1 / norm(ui,2))*((dRciT*Themat+(Rci')*dTheMat) ...
                *(Rci*PiMat*(Rci'))*duihat + (Rci')*Themat*(Rci*PiMat*(Rci'))*(d2uihat-(((ui')*duihat)/(norm(ui,2)^2))*duihat));
dwci = [-dwcxe3(2);  dwcxe3(1);  -dwcxe2(1)];

== matlab function sim_att_dist_obs_tcyb/cal wei agent 1 ==
  data: wi_vec input; wei_1 output; Rei_vec input; wci_vec input
function wei_1 = fcn(wi_vec, Rei_vec, wci_vec)
%%%% 更新姿态角速率误差
iiuav = 1;
wei_1 = wi_vec(:,iiuav) - (Rei_vec(:,:,iiuav)') * wci_vec(:,iiuav);

end

== matlab function sim_att_dist_obs_tcyb/cal wei agent 2 ==
  data: wi_vec input; wei_2 output; Rei_vec input; wci_vec input
function wei_2 = fcn(wi_vec, Rei_vec, wci_vec)
%%%% 更新姿态角速率误差
iiuav = 2;
wei_2 = wi_vec(:,iiuav) - (Rei_vec(:,:,iiuav)') * wci_vec(:,iiuav);

end

== matlab function sim_att_dist_obs_tcyb/cal wei agent 3 ==
  data: wi_vec input; wei_3 output; Rei_vec input; wci_vec input
function wei_3 = fcn(wi_vec, Rei_vec, wci_vec)
%%%% 更新姿态角速率误差
iiuav = 3;
wei_3 = wi_vec(:,iiuav) - (Rei_vec(:,:,iiuav)') * wci_vec(:,iiuav);

end

== matlab function sim_att_dist_obs_tcyb/cal eps_w_hat agent 2 ==
  data: Ji input; Krw input; eps_w_hat_vec input; wi_vec input; d_eps_w_hat_2 output; taui_vec input
function d_eps_w_hat_2 = fcn(Ji, Krw, eps_w_hat_vec, wi_vec, taui_vec)
%%%% 计算扰动观测中间变量
iiuav = 2;
d_eps_w_hat_2 = -Krw * inv(Ji(:,:,iiuav)) * ( eps_w_hat_vec(:,iiuav) + taui_vec(:,iiuav) ...
                                                                        - cal_askew_mat(wi_vec(:,iiuav)) * Ji(:,:,iiuav) * wi_vec(:,iiuav) ) ...
                                                                        - Krw * Krw * inv(Ji(:,:,iiuav)) * wi_vec(:,iiuav);

== matlab function sim_att_dist_obs_tcyb/cal wei agent 4 ==
  data: wi_vec input; wei_4 output; Rei_vec input; wci_vec input
function wei_4 = fcn(wi_vec, Rei_vec, wci_vec)
%%%% 更新姿态角速率误差
iiuav = 4;
wei_4 = wi_vec(:,iiuav) - (Rei_vec(:,:,iiuav)') * wci_vec(:,iiuav);

end

== matlab function sim_att_dist_obs_tcyb/cal wei agent 5 ==
  data: wi_vec input; wei_5 output; Rei_vec input; wci_vec input
function wei_5 = fcn(wi_vec, Rei_vec, wci_vec)
%%%% 更新姿态角速率误差
iiuav = 5;
wei_5 = wi_vec(:,iiuav) - (Rei_vec(:,:,iiuav)') * wci_vec(:,iiuav);

end

== matlab function sim_att_dist_obs_tcyb/choose ksi_est_err 41 ==
  data: x input; y output
function y = fcn(x)
iiuav = 1;
y = x(:,iiuav);

== matlab function sim_att_dist_obs_tcyb/choose ksi_est_err 42 ==
  data: x input; y output
function y = fcn(x)
iiuav = 5;
y = x(:,iiuav);

== matlab function sim_att_dist_obs_tcyb/choose ksi_est_err 52 ==
  data: x input; y output
function y = fcn(x)
iiuav = 1;
y = x(:,iiuav);

== matlab function sim_att_dist_obs_tcyb/choose ksi_est_err 54 ==
  data: x input; y output
function y = fcn(x)
iiuav = 1;
y = x(:,iiuav);

== matlab function sim_att_dist_obs_tcyb/choose ksi_est_err 55 ==
  data: x input; y output
function y = fcn(x)
iiuav = 2;
y = x(:,iiuav);

== matlab function sim_att_dist_obs_tcyb/choose ksi_est_err 56 ==
  data: x input; y output
function y = fcn(x)
iiuav = 3;
y = x(:,iiuav);

== matlab function sim_att_dist_obs_tcyb/choose ksi_est_err 57 ==
  data: x input; y output
function y = fcn(x)
iiuav = 4;
y = x(:,iiuav);

== matlab function sim_att_dist_obs_tcyb/choose ksi_est_err 58 ==
  data: x input; y output
function y = fcn(x)
iiuav = 5;
y = x(:,iiuav);

== matlab function sim_att_dist_obs_tcyb/choose ksi_est_err 59 ==
  data: x input; y output
function y = fcn(x)
iiuav = 1;
y = x(:,iiuav);

== matlab function sim_att_dist_obs_tcyb/choose ksi_est_err 60 ==
  data: x input; y output
function y = fcn(x)
iiuav = 1;
y = x(:,iiuav);

== matlab function sim_att_dist_obs_tcyb/choose ksi_est_err 61 ==
  data: x input; y output
function y = fcn(x)
iiuav = 2;
y = x(:,iiuav);

== matlab function sim_att_dist_obs_tcyb/choose ksi_est_err 62 ==
  data: x input; y output
function y = fcn(x)
iiuav = 2;
y = x(:,iiuav);

== matlab function sim_att_dist_obs_tcyb/choose ksi_est_err 63 ==
  data: x input; y output
function y = fcn(x)
iiuav = 2;
y = x(:,iiuav);

== matlab function sim_att_dist_obs_tcyb/cal eps_w_hat agent 3 ==
  data: Ji input; Krw input; eps_w_hat_vec input; wi_vec input; d_eps_w_hat_3 output; taui_vec input
function d_eps_w_hat_3 = fcn(Ji, Krw, eps_w_hat_vec, wi_vec, taui_vec)
%%%% 计算扰动观测中间变量
iiuav = 3;
d_eps_w_hat_3 = -Krw * inv(Ji(:,:,iiuav)) * ( eps_w_hat_vec(:,iiuav) + taui_vec(:,iiuav) ...
                                                                        - cal_askew_mat(wi_vec(:,iiuav)) * Ji(:,:,iiuav) * wi_vec(:,iiuav) ) ...
                                                                        - Krw * Krw * inv(Ji(:,:,iiuav)) * wi_vec(:,iiuav);

== matlab function sim_att_dist_obs_tcyb/choose ksi_est_err 64 ==
  data: x input; y output
function y = fcn(x)
iiuav = 3;
y = x(:,iiuav);

== matlab function sim_att_dist_obs_tcyb/choose ksi_est_err 65 ==
  data: x input; y output
function y = fcn(x)
iiuav = 3;
y = x(:,iiuav);

== matlab function sim_att_dist_obs_tcyb/choose ksi_est_err 66 ==
  data: x input; y output
function y = fcn(x)
iiuav = 4;
y = x(:,iiuav);

== matlab function sim_att_dist_obs_tcyb/choose ksi_est_err 67 ==
  data: x input; y output
function y = fcn(x)
iiuav = 4;
y = x(:,iiuav);

== matlab function sim_att_dist_obs_tcyb/choose ksi_est_err 68 ==
  data: x input; y output
function y = fcn(x)
iiuav = 5;
y = x(:,iiuav);

== matlab function sim_att_dist_obs_tcyb/choose ksi_est_err 69 ==
  data: x input; y output
function y = fcn(x)
iiuav = 5;
y = x(:,iiuav);

== matlab function sim_att_dist_obs_tcyb/choose ksi_est_err 70 ==
  data: x input; y output
function y = fcn(x)
iiuav = 2;
y = x(:,iiuav);

== matlab function sim_att_dist_obs_tcyb/choose ksi_est_err 71 ==
  data: x input; y output
function y = fcn(x)
iiuav = 3;
y = x(:,iiuav);

== matlab function sim_att_dist_obs_tcyb/choose ksi_est_err 72 ==
  data: x input; y output
function y = fcn(x)
iiuav = 3;
y = x(:,iiuav);

== matlab function sim_att_dist_obs_tcyb/choose ksi_est_err 73 ==
  data: x input; y output
function y = fcn(x)
iiuav = 4;
y = x(:,iiuav);

== matlab function sim_att_dist_obs_tcyb/choose ksi_est_err 74 ==
  data: x input; y output
function y = fcn(x)
iiuav = 4;
y = x(:,iiuav);

== matlab function sim_att_dist_obs_tcyb/choose ksi_est_err 75 ==
  data: x input; y output
function y = fcn(x)
iiuav = 5;
y = x(:,iiuav);

== matlab function sim_att_dist_obs_tcyb/choose ui agent 1 ==
  data: x input; y output
function y = fcn(x)
iiuav = 1;
y = x(:,iiuav);

== matlab function sim_att_dist_obs_tcyb/choose ui agent 2 ==
  data: x input; y output
function y = fcn(x)
iiuav = 2;
y = x(:,iiuav);

== matlab function sim_att_dist_obs_tcyb/choose ui agent 3 ==
  data: x input; y output
function y = fcn(x)
iiuav = 3;
y = x(:,iiuav);

== matlab function sim_att_dist_obs_tcyb/choose ui agent 4 ==
  data: x input; y output
function y = fcn(x)
iiuav = 4;
y = x(:,iiuav);

== matlab function sim_att_dist_obs_tcyb/cal eps_w_hat agent 4 ==
  data: Ji input; Krw input; eps_w_hat_vec input; wi_vec input; d_eps_w_hat_4 output; taui_vec input
function d_eps_w_hat_4 = fcn(Ji, Krw, eps_w_hat_vec, wi_vec, taui_vec)
%%%% 计算扰动观测中间变量
iiuav = 4;
d_eps_w_hat_4 = -Krw * inv(Ji(:,:,iiuav)) * ( eps_w_hat_vec(:,iiuav) + taui_vec(:,iiuav) ...
                                                                        - cal_askew_mat(wi_vec(:,iiuav)) * Ji(:,:,iiuav) * wi_vec(:,iiuav) ) ...
                                                                        - Krw * Krw * inv(Ji(:,:,iiuav)) * wi_vec(:,iiuav);

== matlab function sim_att_dist_obs_tcyb/choose ui agent 5 ==
  data: x input; y output
function y = fcn(x)
iiuav = 5;
y = x(:,iiuav);

== matlab function sim_att_dist_obs_tcyb/combine Fi_S ==
  data: Fi_S_1 input; Fi_S_2 input; Fi_S_3 input; Fi_S_4 input; Fi_S_5 input; Fi_S_vec output
function Fi_S_vec  = fcn(Fi_S_1, Fi_S_2, Fi_S_3, Fi_S_4, Fi_S_5)
%%%% 合并补偿项
Fi_S_vec = zeros(3,5);
Fi_S_vec(:,1) = Fi_S_1(:);
Fi_S_vec(:,2) = Fi_S_2(:);
Fi_S_vec(:,3) = Fi_S_3(:);
Fi_S_vec(:,4) = Fi_S_4(:);
Fi_S_vec(:,5) = Fi_S_5(:);

== matlab function sim_att_dist_obs_tcyb/combine Phi_bar_psi_e ==
  data: Phi_bar_psi_e_node_1 input; Phi_bar_psi_e_node_2 input; Phi_bar_psi_e_node_3 input; Phi_bar_psi_e_node_4 input; Phi_bar_psi_e_node_5 input; Phi_bar_psi_e_vec output
function Phi_bar_psi_e_vec  = fcn(Phi_bar_psi_e_node_1, Phi_bar_psi_e_node_2, Phi_bar_psi_e_node_3, ...
                                                                Phi_bar_psi_e_node_4, Phi_bar_psi_e_node_5)
%%%% 合并姿态误差导数
Phi_bar_psi_e_vec = zeros(3,5);
Phi_bar_psi_e_vec(:,1) = Phi_bar_psi_e_node_1(:);
Phi_bar_psi_e_vec(:,2) = Phi_bar_psi_e_node_2(:);
Phi_bar_psi_e_vec(:,3) = Phi_bar_psi_e_node_3(:);
Phi_bar_psi_e_vec(:,4) = Phi_bar_psi_e_node_4(:);
Phi_bar_psi_e_vec(:,5) = Phi_bar_psi_e_node_5(:);

== matlab function sim_att_dist_obs_tcyb/combine Phi_psi_e ==
  data: Phi_psi_e_node_1 input; Phi_psi_e_node_2 input; Phi_psi_e_node_3 input; Phi_psi_e_node_4 input; Phi_psi_e_node_5 input; Phi_psi_e_vec output
function Phi_psi_e_vec  = fcn(Phi_psi_e_node_1, Phi_psi_e_node_2, Phi_psi_e_node_3, ...
                                                        Phi_psi_e_node_4, Phi_psi_e_node_5)
%%%% 合并姿态误差项
Phi_psi_e_vec = zeros(3,5);
Phi_psi_e_vec(:,1) = Phi_psi_e_node_1(:);
Phi_psi_e_vec(:,2) = Phi_psi_e_node_2(:);
Phi_psi_e_vec(:,3) = Phi_psi_e_node_3(:);
Phi_psi_e_vec(:,4) = Phi_psi_e_node_4(:);
Phi_psi_e_vec(:,5) = Phi_psi_e_node_5(:);

== matlab function sim_att_dist_obs_tcyb/combine Qci Rci ==
  data: Qci_1 input; Qci_vec output; Qci_2 input; Qci_3 input; Qci_4 input; Qci_5 input; Rci_1 input; Rci_2 input; Rci_3 input; Rci_4 input; Rci_5 input; Rci_vec output
function [Qci_vec, Rci_vec] = fcn(Qci_1, Qci_2, Qci_3, Qci_4, Qci_5, ...
                                                            Rci_1, Rci_2, Rci_3, Rci_4, Rci_5)
%%%% 合并四元数和姿态旋转矩阵
Qci_vec = zeros(4,5);
Qci_vec(:,1) = Qci_1(:);
Qci_vec(:,2) = Qci_2(:);
Qci_vec(:,3) = Qci_3(:);
Qci_vec(:,4) = Qci_4(:);
Qci_vec(:,5) = Qci_5(:);

Rci_vec = zeros(3,3,5);
Rci_vec(:,:,1) = Rci_1;
Rci_vec(:,:,2) = Rci_2;
Rci_vec(:,:,3) = Rci_3;
Rci_vec(:,:,4) = Rci_4;
Rci_vec(:,:,5) = Rci_5;

== matlab function sim_att_dist_obs_tcyb/combine Qci Rci1 ==
  data: V_Phi_Rei_1 input; V_Phi_Rei_vec output; V_Phi_Rei_2 input; V_Phi_Rei_3 input; V_Phi_Rei_4 input; V_Phi_Rei_5 input
function V_Phi_Rei_vec = fcn(V_Phi_Rei_1, V_Phi_Rei_2, V_Phi_Rei_3, V_Phi_Rei_4, V_Phi_Rei_5)
%%%% 合并LogSO3空间的辅助姿态误差向量
V_Phi_Rei_vec = [V_Phi_Rei_1(:), V_Phi_Rei_2(:), V_Phi_Rei_3(:), V_Phi_Rei_4(:), V_Phi_Rei_5(:)];

== matlab function sim_att_dist_obs_tcyb/combine Qi Ri ==
  data: Qi_1 input; Qi_vec output; Qi_2 input; Qi_3 input; Qi_4 input; Qi_5 input; Ri_1 input; Ri_2 input; Ri_3 input; Ri_4 input; Ri_5 input; Ri_vec output
function [Qi_vec, Ri_vec] = fcn(Qi_1, Qi_2, Qi_3, Qi_4, Qi_5, ...
                                                        Ri_1, Ri_2, Ri_3, Ri_4, Ri_5)
%%%% 合并四元数和姿态旋转矩阵
Qi_vec = zeros(4,5);
Qi_vec(:,1) = Qi_1(:);
Qi_vec(:,2) = Qi_2(:);
Qi_vec(:,3) = Qi_3(:);
Qi_vec(:,4) = Qi_4(:);
Qi_vec(:,5) = Qi_5(:);

Ri_vec = zeros(3,3,5);
Ri_vec(:,:,1) = Ri_1;
Ri_vec(:,:,2) = Ri_2;
Ri_vec(:,:,3) = Ri_3;
Ri_vec(:,:,4) = Ri_4;
Ri_vec(:,:,5) = Ri_5;

== matlab function sim_att_dist_obs_tcyb/combine S_bar ==
  data: S_bar_node_1 input; S_bar_node_2 input; S_bar_node_3 input; S_bar_node_4 input; S_bar_node_5 input; S_bar_vec output
function S_bar_vec  = fcn(S_bar_node_1, S_bar_node_2, S_bar_node_3, ...
                                                S_bar_node_4, S_bar_node_5)
%%%% 合并辅助滑模面
S_bar_vec = zeros(3,5);
S_bar_vec(:,1) = S_bar_node_1(:);
S_bar_vec(:,2) = S_bar_node_2(:);
S_bar_vec(:,3) = S_bar_node_3(:);
S_bar_vec(:,4) = S_bar_node_4(:);
S_bar_vec(:,5) = S_bar_node_5(:);

== matlab function sim_att_dist_obs_tcyb/combine Si ==
  data: Si_1 input; Si_2 input; Si_3 input; Si_4 input; Si_5 input; Si_vec output
function Si_vec  = fcn(Si_1, Si_2, Si_3, Si_4, Si_5)
%%%% 合并滑模面
Si_vec = zeros(3,5);
Si_vec(:,1) = Si_1(:);
Si_vec(:,2) = Si_2(:);
Si_vec(:,3) = Si_3(:);
Si_vec(:,4) = Si_4(:);
Si_vec(:,5) = Si_5(:);

== matlab function sim_att_dist_obs_tcyb/combine Si_squ_beta_w_1 ==
  data: Si_squ_beta_w_1_node_1 input; Si_squ_beta_w_1_node_2 input; Si_squ_beta_w_1_node_3 input; Si_squ_beta_w_1_node_4 input; Si_squ_beta_w_1_node_5 input; Si_squ_beta_w_1_vec output
function Si_squ_beta_w_1_vec  = fcn(Si_squ_beta_w_1_node_1, Si_squ_beta_w_1_node_2, Si_squ_beta_w_1_node_3, ...
                                                                    Si_squ_beta_w_1_node_4, Si_squ_beta_w_1_node_5)
%%%% 合并误差幂次项
Si_squ_beta_w_1_vec = zeros(3,5);
Si_squ_beta_w_1_vec(:,1) = Si_squ_beta_w_1_node_1(:);
Si_squ_beta_w_1_vec(:,2) = Si_squ_beta_w_1_node_2(:);
Si_squ_beta_w_1_vec(:,3) = Si_squ_beta_w_1_node_3(:);
Si_squ_beta_w_1_vec(:,4) = Si_squ_beta_w_1_node_4(:);
Si_squ_beta_w_1_vec(:,5) = Si_squ_beta_w_1_node_5(:);

== matlab function sim_att_dist_obs_tcyb/cal eps_w_hat agent 5 ==
  data: Ji input; Krw input; eps_w_hat_vec input; wi_vec input; d_eps_w_hat_5 output; taui_vec input
function d_eps_w_hat_5 = fcn(Ji, Krw, eps_w_hat_vec, wi_vec, taui_vec)
%%%% 计算扰动观测中间变量
iiuav = 5;
d_eps_w_hat_5 = -Krw * inv(Ji(:,:,iiuav)) * ( eps_w_hat_vec(:,iiuav) + taui_vec(:,iiuav) ...
                                                                        - cal_askew_mat(wi_vec(:,iiuav)) * Ji(:,:,iiuav) * wi_vec(:,iiuav) ) ...
                                                                        - Krw * Krw * inv(Ji(:,:,iiuav)) * wi_vec(:,iiuav);

== matlab function sim_att_dist_obs_tcyb/combine Si_squ_beta_w_2 ==
  data: Si_squ_beta_w_2_node_1 input; Si_squ_beta_w_2_node_2 input; Si_squ_beta_w_2_node_3 input; Si_squ_beta_w_2_node_4 input; Si_squ_beta_w_2_node_5 input; Si_squ_beta_w_2_vec output
function Si_squ_beta_w_2_vec  = fcn(Si_squ_beta_w_2_node_1, Si_squ_beta_w_2_node_2, Si_squ_beta_w_2_node_3, ...
                                                                    Si_squ_beta_w_2_node_4, Si_squ_beta_w_2_node_5)
%%%% 合并误差幂次项
Si_squ_beta_w_2_vec = zeros(3,5);
Si_squ_beta_w_2_vec(:,1) = Si_squ_beta_w_2_node_1(:);
Si_squ_beta_w_2_vec(:,2) = Si_squ_beta_w_2_node_2(:);
Si_squ_beta_w_2_vec(:,3) = Si_squ_beta_w_2_node_3(:);
Si_squ_beta_w_2_vec(:,4) = Si_squ_beta_w_2_node_4(:);
Si_squ_beta_w_2_vec(:,5) = Si_squ_beta_w_2_node_5(:);

== matlab function sim_att_dist_obs_tcyb/combine V_Phi_Rei_squ_2p ==
  data: V_Phi_Rei_squ_2p_node_1 input; V_Phi_Rei_squ_2p_node_2 input; V_Phi_Rei_squ_2p_node_3 input; V_Phi_Rei_squ_2p_node_4 input; V_Phi_Rei_squ_2p_node_5 input; V_Phi_Rei_squ_2p_vec output
function V_Phi_Rei_squ_2p_vec  = fcn(V_Phi_Rei_squ_2p_node_1, V_Phi_Rei_squ_2p_node_2, V_Phi_Rei_squ_2p_node_3, ...
                                                                        V_Phi_Rei_squ_2p_node_4, V_Phi_Rei_squ_2p_node_5)
%%%% 合并姿态误差指数坐标
V_Phi_Rei_squ_2p_vec = zeros(3,5);
V_Phi_Rei_squ_2p_vec(:,1) = V_Phi_Rei_squ_2p_node_1(:);
V_Phi_Rei_squ_2p_vec(:,2) = V_Phi_Rei_squ_2p_node_2(:);
V_Phi_Rei_squ_2p_vec(:,3) = V_Phi_Rei_squ_2p_node_3(:);
V_Phi_Rei_squ_2p_vec(:,4) = V_Phi_Rei_squ_2p_node_4(:);
V_Phi_Rei_squ_2p_vec(:,5) = V_Phi_Rei_squ_2p_node_5(:);
